simulink model "OpAmpOscillator"  (R2022b)
settings: Solver=VariableStepAuto  StartTime=0.0  StopTime=(1/10e9)*5  RelTol=1e-3
settings Model: Creator=minar  LastModifiedBy=minar

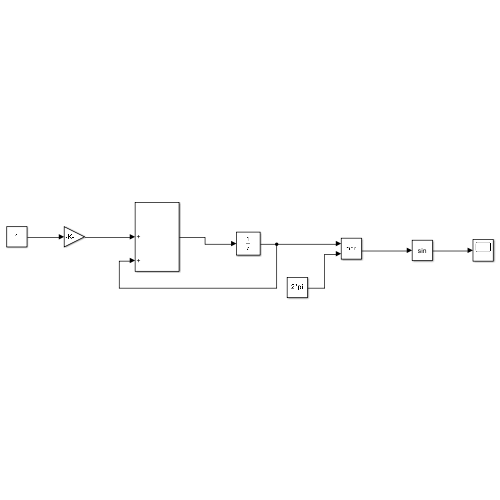
[thumbnail: Simulink's stored preview of the top-level diagram]
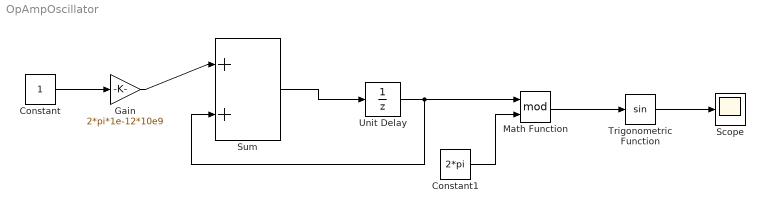
== system OpAmpOscillator ==
  Constant : Constant
  Constant1 : Constant  Value=2*pi
  Gain : Gain  Gain=2*pi*1e-12*10e9
  Math Function : Math  Operator=mod
  Scope : Scope
  Sum : Sum  Inputs=|++
  Trigonometric Function : Trigonometry
  Unit Delay : UnitDelay  SampleTime=1e-12  HasFrameUpgradeWarning=on
  wires:
  Constant/1 -> Gain/1
  Gain/1 -> Sum/1
  Sum/1 -> Unit Delay/1
  Unit Delay/1 -> Sum/2, Math Function/1
  Constant1/1 -> Math Function/2
  Math Function/1 -> Trigonometric Function/1
  Trigonometric Function/1 -> Scope/1
